simulink model "hw5"  (R2019a)
settings: Solver=VariableStepAuto  StartTime=0.0  StopTime=10.0  RelTol=1e-3
settings Model: Creator=sumli  LastModifiedBy=sumli

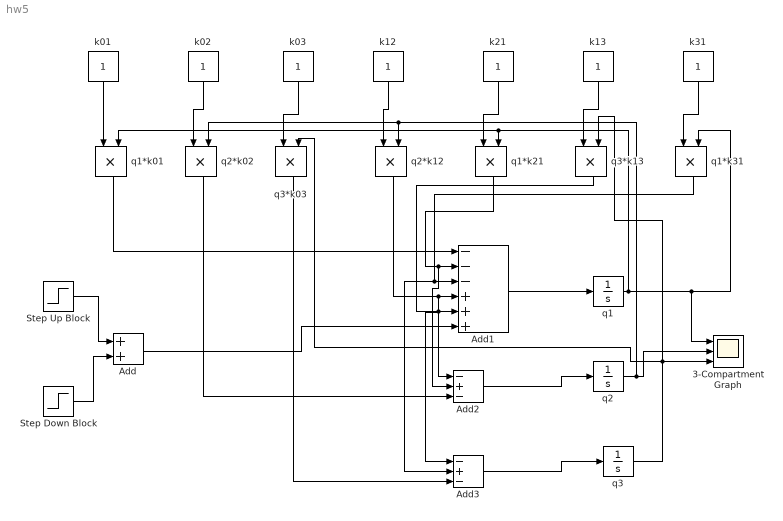
== system hw5 ==
  3-Compartment Graph : Scope  NumInputPorts=3
  Add : Sum
  Add1 : Sum  Inputs=---+++
  Add2 : Sum  Inputs=-+-
  Add3 : Sum  Inputs=-+-
  Step Down Block : Step  Time=1.000001  After=-1000000  SampleTime=0
  Step Up Block : Step  After=1000000  SampleTime=0
  k01 : Constant
  k02 : Constant
  k03 : Constant
  k{12..13,21,31} (4 alike) : Constant
  q1 : Integrator
  q1*k01 : Product
  q1*k21 : Product
  q1*k31 : Product
  q2 : Integrator
  q2*k02 : Product
  q2*k12 : Product
  q3 : Integrator
  q3*k03 : Product
  q3*k13 : Product
  wires:
  q1/1 -> q1*k21/2, q1*k01/2, q1*k31/2, 3-Compartment Graph/1
  q2/1 -> q2*k12/2, q2*k02/2, 3-Compartment Graph/2
  q3/1 -> q3*k03/2, 3-Compartment Graph/3, q3*k13/2
  Step Up Block/1 -> Add/1
  Step Down Block/1 -> Add/2
  Add/1 -> Add1/6
  k01/1 -> q1*k01/1
  Add1/1 -> q1/1
  Add2/1 -> q2/1
  Add3/1 -> q3/1
  k02/1 -> q2*k02/1
  k03/1 -> q3*k03/1
  k12/1 -> q2*k12/1
  k21/1 -> q1*k21/1
  k13/1 -> q3*k13/1
  k31/1 -> q1*k31/1
  q1*k01/1 -> Add1/1
  q1*k21/1 -> Add2/2, Add1/2
  q1*k31/1 -> Add3/2, Add1/3
  q2*k12/1 -> Add2/1, Add1/4
  q3*k13/1 -> Add3/1, Add1/5
  q2*k02/1 -> Add2/3
  q3*k03/1 -> Add3/3
